simulink model "Player"  (R2012b)
settings: Solver=ode1  StartTime=0.0  StopTime=inf  FixedStep=0.002  RelTol=1e-3
settings Model: ExtModeTrigDuration=5000  Creator=anzhuan  LastModifiedBy=anzhuan
settings SolverCC: PositivePriorityOrder=on
settings RTWCC: SystemTargetFile=quarc_win64.tlc  TemplateMakefile=quarc_default_tmf  Description=QUARC Win64 Target  ProcessScript=quarc_win64_make_rtw_hook
settings STFCustomTargetCC: TargetPreCompLibLocation=C:\PROGRA~3\QUARC\lib\2012b\win64\release  CodeReplacementLibrary=ANSI_C  GeneratePreprocessorConditionals=Disable all  CombineOutputUpdateFcns=on  GRTInterface=off  SystemTargetFile=quarc_win64.tlc
settings GRTTargetCC: TargetPreCompLibLocation=C:\PROGRA~3\QUARC\lib\2012b\win64\release  ParMdlRefBuildCompliant=off  CompOptLevelCompliant=off  ConcurrentExecutionCompliant=off  MatFileLogging=off  ExtMode=on  ExtModeMexFile=quarc_comm

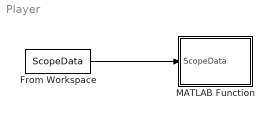
== system Player ==
  From Workspace : FromWorkspace  VariableName=ScopeData  OutDataTypeStr=double
  MATLAB Function : MATLAB Function  TreatAsAtomicUnit=on
  wires:
  From Workspace/1 -> MATLAB Function/1(ScopeData)

== matlab function Player/MATLAB Function ==
  data: ScopeData input
function ReplayScope(ScopeData)
%UNTITLED Summary of this function goes here
%   Detailed explanation goes here
A = [0 0 0];
B = [0 0 -1];
C = [0 6 -1];
D = [0 6 0];
E = [0 8 0];
F = [0 0 0];
G = [0 12 0];

[m,n] = size(ScopeData);
    for i = 1:m
        theta1 = ScopeData(i,2);
        theta2 = ScopeData(i,3);
        
        A1 = TRANS0_1(A,theta1);
        B1 = TRANS0_1(B,theta1);
        C1 = TRANS0_1(C,theta1);
        D1 = TRANS0_1(D,theta1);
        E1 = TRANS0_1(E,theta1);
        
        F2 = TRANS1_2(F,theta2);
        G2 = TRANS1_2(G,theta2);
        F1 = TRANS0_1(F2,theta1);
        G1 = TRANS0_1(G2,theta1);
        
            M = [A1.',B1.',C1.',D1.',E1.'];
            X1 = M(1,:);
            Y1 = M(2,:);
            Z1 = M(3,:);
            
            N = [F1.',G1.'];
            X2 = N(1,:);
            Y2 = N(2,:);
            Z2 = N(3,:);
            
            plot3(X1,Y1,Z1,'r-');
            plot3(X2,Y2,Z2,'b-');
            axis([-15 15 -15 15 -15 15]);
    end
end
